simulink model "Shuttle_Orbiter_FDM"  (R2013b)
settings: Solver=ode45  StartTime=0.0  StopTime=1000  RelTol=1e-3
values from neighbouring files (symbols this model uses):
  b = 23.79    [Orbite_InitialParamaters.m]
  c = 12.06    [Orbite_InitialParamaters.m]
  CD_alpha_mach = [0.11425	0.11975	0.13521	0.16 ... (first row only)    [Aerodynamics.m]
  CD_dbf = [0.0135	0.00959	0.0059	0.00242	-0.0005	0.00005	0.0006	0.0006 ... (first row only)    [Aerodynamics.m]
  CD_de = [0.1526	0.113	0.0796	0.0499	0.0176	-0.0262	-0.0837	-0.1391 ... (first row only)    [Aerodynamics.m]
  CDda = 0    [Aerodynamics.m]
  CDdr = 0    [Aerodynamics.m]
  CDdsb = 0.1    [Aerodynamics.m]
  CG = [1080.0 0.0 370.0]    [Orbite_InitialParamaters.m]
  CL0 = -0.05    [Aerodynamics.m]
  CL_alpha_mach = [-0.5028	-0.51097	-0.52957	-0.58454	-0.59773	-0.61005	-0.62831	-0.65514	-0.65616 ... (first row only)    [Aerodynamics.m]
  Cl_beta = [  0	0	0	0	0	0	0	0 ... (first row only)    [Aerodynamics.m]
  CLalpha = 0.05    [Aerodynamics.m]
  CLalphadot = 0    [Aerodynamics.m]
  Clbeta = -0.001    [Aerodynamics.m]
  Clda = 0.0001    [Aerodynamics.m]
  CLde = 0.02    [Aerodynamics.m]
  CLdf = 0.003    [Aerodynamics.m]
  Cldr = 0.00002    (= 2e-05)    [Aerodynamics.m]
  Cldsb = 0.000008    (= 8e-06)    [Aerodynamics.m]
  Clp = -0.003    [Aerodynamics.m]
  CLq = 0    [Aerodynamics.m]
  Clr = 0.006    [Aerodynamics.m]
  Cm0 = 0.036    [Aerodynamics.m]
  Cma = -0.012    [Aerodynamics.m]
  Cmde = -0.087    [Aerodynamics.m]
  Cmdf = -0.0017    [Aerodynamics.m]
  Cmdsb = 0.006    [Aerodynamics.m]
  Cmq = 0.058    [Aerodynamics.m]
  Cnbeta = 0.0016    [Aerodynamics.m]
  Cnda = 0.00005    (= 5e-05)    [Aerodynamics.m]
  Cndr = 0.000006    (= 6e-06)    [Aerodynamics.m]
  Cndsb = 0    [Aerodynamics.m]
  Cnp = -0.0046    [Aerodynamics.m]
  Cnr = -0.005    [Aerodynamics.m]
  CP = [1080.0 0.0 370.0]    [Orbite_InitialParamaters.m]
  CY_da = [0.00106	0.00048 	-0.00002	-0.0005     -0.0008 	-0.00102	-0.00116	-0.0014     -0.00125 ... (first row only)    [Aerodynamics.m]
  CY_de = [  -0.0004	0        0.0004	0.00096	0.0012	0.00111	0.0007	0.00045 ... (first row only)    [Aerodynamics.m]
  CY_dr = [   0.00315	0.0031	0.003	0.0029	0.00275	0.00262	0.0026	0.0026 ... (first row only)    [Aerodynamics.m]
  CY_dsb = [  0.00015 0.00007 0.00015 0.0004 0.0008	0.00133	0.002	0.0026 ... (first row only)    [Aerodynamics.m]
  CYbeta = -0.02    [Aerodynamics.m]
  CYda = 0.003    [Aerodynamics.m]
  CYdr = -0.00002    (= -2e-05)    [Aerodynamics.m]
  CYp = 0    [Aerodynamics.m]
  CYr = 0    [Aerodynamics.m]
  GlideSlopeInitial = -20    [Orbite_InitialParamaters.m]
  h_Initial = 3187+0    (= 3187)    [Orbite_InitialParamaters.m]
  heading0 = 117.5    [Orbite_InitialParamaters.m]
  HglideOrbiter = GligeSlope(:,2)    [Orbite_InitialParamaters.m]
  Iyy = 8729397    [Orbite_InitialParamaters.m]
  LongLat0 = [initial_deg(2); initial_deg(1)]    [Orbite_InitialParamaters.m]
  mass = 83000    [Orbite_InitialParamaters.m]
  runway_alt = 1    [Orbite_InitialParamaters.m]
  runway_deg = dms2degrees(runway_dms_FG)    [Orbite_InitialParamaters.m]
  S = 249.91    [Orbite_InitialParamaters.m]
  Tc = 1/25    (= 0.04)    [Orbite_InitialParamaters.m]
  XglideOrbiter = GligeSlope(:,1)    [Orbite_InitialParamaters.m]
undefined symbols (not defined in the file or in its folder): Earth, Receive, Send, WGS84
libraries: aerolibconvert2 x17, aerolibfltsims x5, simulink x3, aerolibasang x3, aerolibtransform2 x2, aerolibobsolete x1, aerolib6dof2 x1, aerolibatmos2 x1, aerolibgravity2 x1
(part 2 of 2)

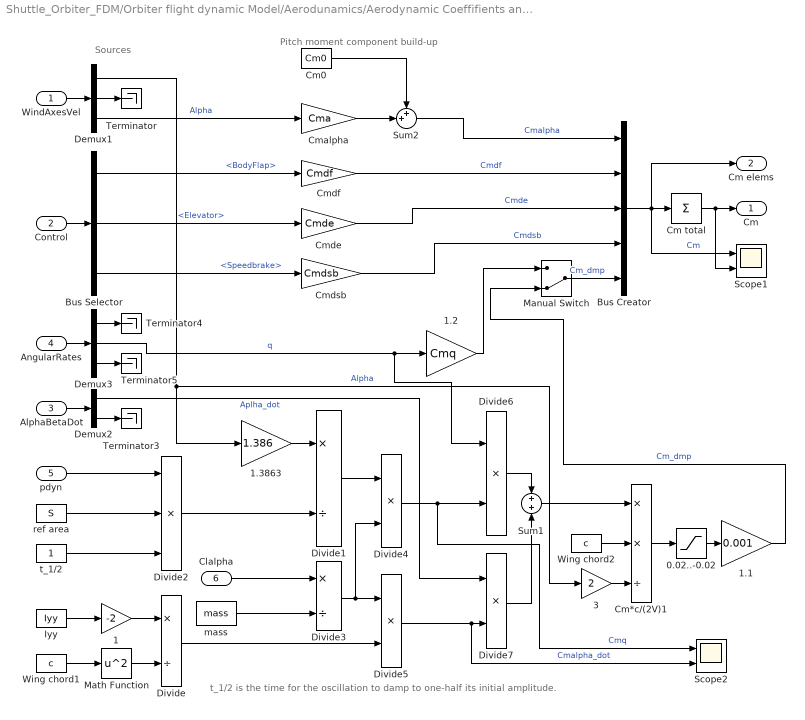
== system Shuttle_Orbiter_FDM/Orbiter flight dynamic Model/Aerodunamics/Aerodynamic Coeffifients and Loads/Pitch Moment Coefficient ==
  note: t_1/2 is the time for the oscillation to damp to one-half its initial amplitude.
  note: Sources
  note: Pitch moment component build-up
  WindAxesVel : Inport
  Control : Inport  Port=2
  AlphaBetaDot : Inport  Port=3
  AngularRates : Inport  Port=4
  pdyn : Inport  Port=5
  Clalpha : Inport  Port=6
  0.02..-0.02 : Saturate  UpperLimit=0.02  LowerLimit=-0.02
  1 : Gain  Gain=-2  SaturateOnIntegerOverflow=on  OutDataTypeStr=Inherit: Same as input  ParamDataTypeStr=Inherit: Same as input
  1.1 : Gain  Gain=0.001  SaturateOnIntegerOverflow=on  OutDataTypeStr=Inherit: Same as input  ParamDataTypeStr=Inherit: Same as input
  1.2 : Gain  Gain=Cmq  SaturateOnIntegerOverflow=on  OutDataTypeStr=Inherit: Same as input  ParamDataTypeStr=Inherit: Same as input
  1.3863 : Gain  Gain=1.386  SaturateOnIntegerOverflow=on  OutDataTypeStr=Inherit: Same as input  ParamDataTypeStr=Inherit: Same as input
  3 : Gain  Gain=2  SaturateOnIntegerOverflow=on  OutDataTypeStr=Inherit: Same as input  ParamDataTypeStr=Inherit: Same as input
  Bus Creator : BusCreator  Inputs=5
  Bus Selector : BusSelector  OutputSignals=BodyFlap,Elevator,Speedbrake
  Cm total : Sum  Inputs=+
  Cm*c/(2V)1 : Product  Inputs=**/  SaturateOnIntegerOverflow=on  InputSameDT=on  OutDataTypeStr=Inherit: Same as first input
  Cm0 : Constant  Value=Cm0  SampleTime=Tc
  Cmalpha : Gain  Gain=Cma  SaturateOnIntegerOverflow=on  OutDataTypeStr=Inherit: Same as input  ParamDataTypeStr=Inherit: Same as input
  Cmde : Gain  Gain=Cmde  SaturateOnIntegerOverflow=on  OutDataTypeStr=Inherit: Same as input  ParamDataTypeStr=Inherit: Same as input
  Cmdf : Gain  Gain=Cmdf  SaturateOnIntegerOverflow=on  OutDataTypeStr=Inherit: Same as input  ParamDataTypeStr=Inherit: Same as input
  Cmdsb : Gain  Gain=Cmdsb  SaturateOnIntegerOverflow=on  OutDataTypeStr=Inherit: Same as input  ParamDataTypeStr=Inherit: Same as input
  Demux1 : Demux  Outputs=3
  Demux2 : Demux  Outputs=2
  Demux3 : Demux  Outputs=3
  Divide : Product  Inputs=*/
  Divide1 : Product  Inputs=*/
  Divide2 : Product  Inputs=3
  Divide3 : Product  Inputs=*/
  Divide{4..7} (4 alike) : Product  Inputs=**
  Iyy : Constant  Value=Iyy  SampleTime=Tc
  Manual Switch : ManualSwitch  CurrentSetting=0
  Math Function : Math  Operator=square  SaturateOnIntegerOverflow=on
  Scope1 : Scope  NumInputPorts=2
      settings: ShowLegends=on  YMin=-0.003~-0.003  YMax=0.003~0.003
  Scope2 : Scope  NumInputPorts=2
      settings: ShowLegends=on  YMin=2.6e-11~-0.0715  YMax=2.925e-11~-0.064  SaveName=ScopeData2
  Sum1 : Sum  SaturateOnIntegerOverflow=on  InputSameDT=on  OutDataTypeStr=Inherit: Same as first input
  Sum2 : Sum  Inputs=++|  SaturateOnIntegerOverflow=on  InputSameDT=on  OutDataTypeStr=Inherit: Same as first input
  Terminator{,3..5} (4 alike) : Terminator
  Wing chord1 : Constant  Value=c  SampleTime=Tc
  Wing chord2 : Constant  Value=c  SampleTime=Tc
  mass : Constant  Value=mass  SampleTime=Tc
  ref area : Constant  Value=S  SampleTime=Tc
  t_1/2 : Constant  SampleTime=Tc
  Cm : Outport
  Cm elems : Outport  Port=2
  wires:
  WindAxesVel/1 -> Demux1/1
  Demux1/1 -> 1.3863/1, 3/1  "Alpha"
  Demux1/2 -> Terminator/1
  Demux1/3 -> Cmalpha/1  "Alpha"
  Control/1 -> Bus Selector/1
  Demux2/1 -> Divide7/1  "Aplha_dot"
  Demux2/2 -> Terminator3/1
  AlphaBetaDot/1 -> Demux2/1
  AngularRates/1 -> Demux3/1
  Demux3/1 -> Terminator4/1
  Demux3/2 -> Divide6/1, 1.2/1  "q"
  Demux3/3 -> Terminator5/1
  Cm0/1 -> Sum2/1
  Cmalpha/1 -> Sum2/2
  Cmdf/1 -> Bus Creator/2  "Cmdf"
  Cmde/1 -> Bus Creator/3  "Cmde"
  Bus Selector/1 -> Cmdf/1  "<BodyFlap>"
  Bus Selector/2 -> Cmde/1  "<Elevator>"
  Bus Selector/3 -> Cmdsb/1  "<Speedbrake>"
  Cmdsb/1 -> Bus Creator/4  "Cmdsb"
  Bus Creator/1 -> Scope1/1, Cm total/1, Cm elems/1  "Cm"
  Iyy/1 -> 1/1
  Wing chord1/1 -> Math Function/1
  1/1 -> Divide/1
  Math Function/1 -> Divide/2
  1.3863/1 -> Divide1/1
  pdyn/1 -> Divide2/1
  ref area/1 -> Divide2/2
  t_1/2/1 -> Divide2/3
  Divide2/1 -> Divide1/2
  mass/1 -> Divide3/2
  Divide/1 -> Divide5/2
  Divide1/1 -> Divide4/1
  0.02..-0.02/1 -> 1.1/1
  Cm total/1 -> Scope1/2, Cm/1
  Divide3/1 -> Divide4/2, Divide5/1
  Divide4/1 -> Scope2/1, Divide6/2  "Cmq"
  Divide5/1 -> Scope2/2, Divide7/2  "Cmalpha_dot"
  Divide7/1 -> Sum1/2
  Divide6/1 -> Sum1/1
  3/1 -> Cm*c/(2V)1/3
  Wing chord2/1 -> Cm*c/(2V)1/2
  Sum1/1 -> Cm*c/(2V)1/1
  Cm*c/(2V)1/1 -> 0.02..-0.02/1
  Sum2/1 -> Bus Creator/1  "Cmalpha"
  1.1/1 -> Manual Switch/2  "Cm_dmp"
  Clalpha/1 -> Divide3/1
  Manual Switch/1 -> Bus Creator/5  "Cm_dmp"
  1.2/1 -> Manual Switch/1

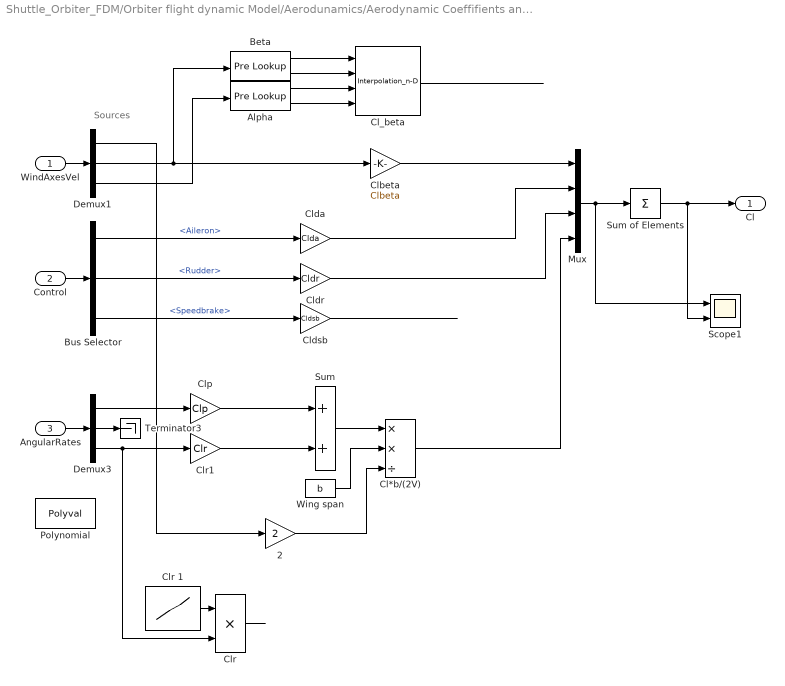
== system Shuttle_Orbiter_FDM/Orbiter flight dynamic Model/Aerodunamics/Aerodynamic Coeffifients and Loads/Roll Moment Coefficient ==
  note: Sources
  WindAxesVel : Inport
  Control : Inport  Port=2
  AngularRates : Inport  Port=3
  2 : Gain  Gain=2  SaturateOnIntegerOverflow=on  OutDataTypeStr=Inherit: Same as input  ParamDataTypeStr=Inherit: Same as input
  Alpha : PreLookup  BreakpointsData=|  ExtrapMethod=Linear
      | [-10 -5  0	5 10  15 20 25
      | ]
  Beta : PreLookup  BreakpointsData=|  ExtrapMethod=Linear
      | [0
      | 1
      | 2
      | 4
      | 6
      | 8
      | 10
      | ]
  Bus Selector : BusSelector  OutputSignals=Aileron,Rudder,Speedbrake
  Cl*b/(2V) : Product  Inputs=**/  SaturateOnIntegerOverflow=on  InputSameDT=on  OutDataTypeStr=Inherit: Same as first input
  "Cl_beta " : Interpolation_n-D  Table=Cl_beta  InternalRulePriority=Speed
  Clbeta : Gain  Gain=Clbeta  SaturateOnIntegerOverflow=on  OutDataTypeStr=Inherit: Same as input  ParamDataTypeStr=Inherit: Same as input
  Clda : Gain  Gain=Clda  SaturateOnIntegerOverflow=on  OutDataTypeStr=Inherit: Same as input  ParamDataTypeStr=Inherit: Same as input
  Cldr : Gain  Gain=Cldr  SaturateOnIntegerOverflow=on  OutDataTypeStr=Inherit: Same as input  ParamDataTypeStr=Inherit: Same as input
  Cldsb : Gain  Gain=Cldsb  SaturateOnIntegerOverflow=on  OutDataTypeStr=Inherit: Same as input  ParamDataTypeStr=Inherit: Same as input
  Clp : Gain  Gain=Clp  SaturateOnIntegerOverflow=on  OutDataTypeStr=Inherit: Same as input  ParamDataTypeStr=Inherit: Same as input
  Clr : Product  SaturateOnIntegerOverflow=on  InputSameDT=on  OutDataTypeStr=Inherit: Same as first input
  Clr 1 : Lookup_n-D  NumberOfTableDimensions=1  BreakpointsForDimension1=|  Table=|  InternalRulePriority=Speed  RndMeth=Simplest  InputSameDT=on
      BreakpointsForDimension1=|
      | [0
      | 10
      | 20
      | 30
      | 40
      | 50
      | ]
      Table=|
      | [0.125
      | 0.188
      | 0.225
      | 0.1
      | 0.075
      | 0.007
      | ]
  Clr1 : Gain  Gain=Clr  SaturateOnIntegerOverflow=on  OutDataTypeStr=Inherit: Same as input  ParamDataTypeStr=Inherit: Same as input
  Demux1 : Demux  Outputs=3
  Demux3 : Demux  Outputs=3
  Mux : Mux
  Polynomial : Polyval  Coefs=[ +2.081618890e-019, -1.441693666e-014, +4.719686976e-010, -8.536869453e-006, +1.621573104e-001, -8.087801117e+001 ]
  Scope1 : Scope  NumInputPorts=2
      settings: ShowLegends=on  YMin=-0.005~-0.005  YMax=0.008~0.008  SaveName=ScopeData3
  Sum : Sum  SaturateOnIntegerOverflow=on  InputSameDT=on  OutDataTypeStr=Inherit: Same as first input
  Sum of Elements : Sum  Inputs=+
  Terminator3 : Terminator
  Wing span : Constant  Value=b  SampleTime=Tc
  Cl : Outport
  wires:
  Clp/1 -> Sum/1
  Clr/1 -> ?
  Sum/1 -> Cl*b/(2V)/1
  Wing span/1 -> Cl*b/(2V)/2
  WindAxesVel/1 -> Demux1/1
  Demux1/1 -> 2/1
  Demux1/2 -> Beta/1, Clbeta/1
  Demux1/3 -> Alpha/1
  AngularRates/1 -> Demux3/1
  Demux3/1 -> Clp/1
  Demux3/2 -> Terminator3/1
  Demux3/3 -> Clr1/1, Clr/2
  Clbeta/1 -> Mux/1
  Clda/1 -> Mux/2
  Cldr/1 -> Mux/3
  Cl*b/(2V)/1 -> Mux/4
  2/1 -> Cl*b/(2V)/3
  Control/1 -> Bus Selector/1
  Bus Selector/1 -> Clda/1  "<Aileron>"
  Bus Selector/2 -> Cldr/1  "<Rudder>"
  Alpha/1 -> "Cl_beta "/3
  Alpha/2 -> "Cl_beta "/4
  Beta/1 -> "Cl_beta "/1
  Beta/2 -> "Cl_beta "/2
  "Cl_beta "/1 -> ?
  Bus Selector/3 -> Cldsb/1  "<Speedbrake>"
  Cldsb/1 -> ?
  Clr1/1 -> Sum/2
  Clr 1/1 -> Clr/1
  Mux/1 -> Sum of Elements/1, Scope1/1
  Sum of Elements/1 -> Cl/1, Scope1/2

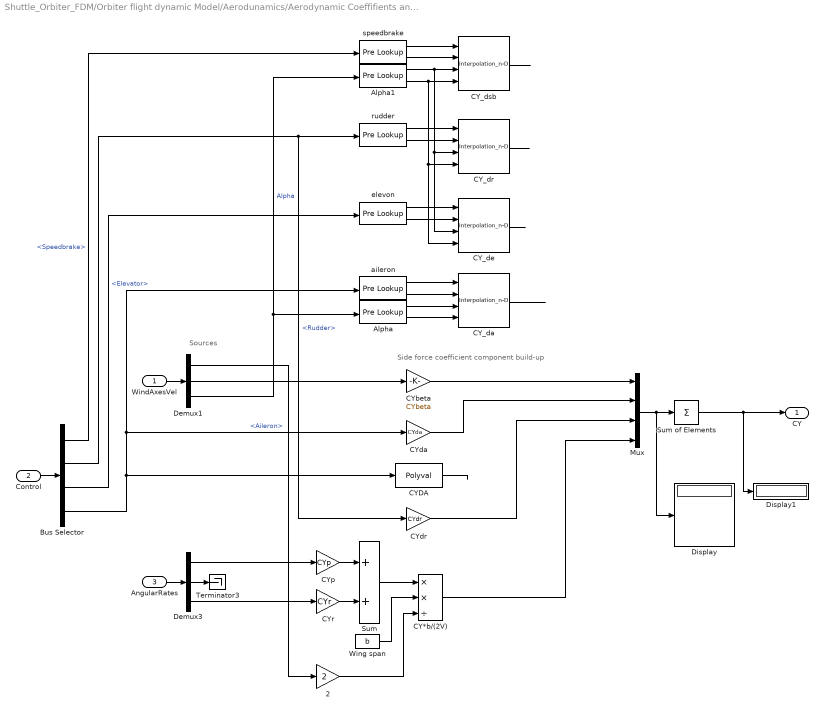
== system Shuttle_Orbiter_FDM/Orbiter flight dynamic Model/Aerodunamics/Aerodynamic Coeffifients and Loads/Side Force Coefficient ==
  note: Sources
  note: Side force coefficient component build-up
  WindAxesVel : Inport
  Control : Inport  Port=2
  AngularRates : Inport  Port=3
  2 : Gain  Gain=2  SaturateOnIntegerOverflow=on  OutDataTypeStr=Inherit: Same as input  ParamDataTypeStr=Inherit: Same as input
  Alpha : PreLookup  BreakpointsData=|  ExtrapMethod=Linear
      | [-10 -5  0	5 10 13 15 20 25
      | ]
  Alpha1 : PreLookup  BreakpointsData=|  ExtrapMethod=Linear
      | [-10 -5  0	5 10  15 20 25
      | ]
  Bus Selector : BusSelector  OutputSignals=Speedbrake,Rudder,Elevator,Aileron
  CY*b/(2V) : Product  Inputs=**/  SaturateOnIntegerOverflow=on  InputSameDT=on  OutDataTypeStr=Inherit: Same as first input
  "CYDA " : Polyval  Coefs=[0.000004 000001 -0.004]
  CY_da : Interpolation_n-D  Table=CY_da  InternalRulePriority=Speed
  CY_de : Interpolation_n-D  Table=CY_de  InternalRulePriority=Speed
  CY_dr : Interpolation_n-D  Table=CY_dr  InternalRulePriority=Speed
  CY_dsb : Interpolation_n-D  Table=CY_dsb  InternalRulePriority=Speed
  CYbeta : Gain  Gain=CYbeta  SaturateOnIntegerOverflow=on  OutDataTypeStr=Inherit: Same as input  ParamDataTypeStr=Inherit: Same as input
  "CYda " : Gain  Gain=CYda  SaturateOnIntegerOverflow=on  OutDataTypeStr=Inherit: Same as input  ParamDataTypeStr=Inherit: Same as input
  CYdr : Gain  Gain=CYdr  SaturateOnIntegerOverflow=on  OutDataTypeStr=Inherit: Same as input  ParamDataTypeStr=Inherit: Same as input
  CYp : Gain  Gain=CYp  SaturateOnIntegerOverflow=on  OutDataTypeStr=Inherit: Same as input  ParamDataTypeStr=Inherit: Same as input
  CYr : Gain  Gain=CYr  SaturateOnIntegerOverflow=on  OutDataTypeStr=Inherit: Same as input  ParamDataTypeStr=Inherit: Same as input
  Demux1 : Demux  Outputs=3
  Demux3 : Demux  Outputs=3
  Display : Display
  Display1 : Display
  Mux : Mux
  Sum : Sum  SaturateOnIntegerOverflow=on  InputSameDT=on  OutDataTypeStr=Inherit: Same as first input
  Sum of Elements : Sum  Inputs=+
  Terminator3 : Terminator
  Wing span : Constant  Value=b  SampleTime=Tc
  aileron : PreLookup  BreakpointsData=|  ExtrapMethod=Linear
      | [-30
      | -25
      | -20
      | -15
      | -10
      | -5
      | 0
      | 5
      | 10
      | 15]
  elevon : PreLookup  BreakpointsData=|  ExtrapMethod=Linear
      | [-30
      | -25
      | -20
      | -15
      | -10
      | -5
      | 0
      | 5
      | 10
      | 15
      | ]
  rudder : PreLookup  BreakpointsData=|  ExtrapMethod=Linear
      | [0
      | 7.5
      | 15
      | 25
      | 35
      | 45
      | 55
      | 70
      | 87.2
      | ]
  speedbrake : PreLookup  BreakpointsData=|  ExtrapMethod=Linear
      | [0
      | 15
      | 25
      | 35
      | 45
      | 55
      | 70
      | 87.2
      | ]
  CY : Outport
  wires:
  CYp/1 -> Sum/1
  CYr/1 -> Sum/2
  Sum/1 -> CY*b/(2V)/1
  Wing span/1 -> CY*b/(2V)/2
  WindAxesVel/1 -> Demux1/1
  Demux1/1 -> 2/1
  Demux1/2 -> CYbeta/1
  Control/1 -> Bus Selector/1
  AngularRates/1 -> Demux3/1
  Demux3/1 -> CYp/1
  Demux3/2 -> Terminator3/1
  Demux3/3 -> CYr/1
  CYbeta/1 -> Mux/1
  "CYda "/1 -> Mux/2
  CYdr/1 -> Mux/3
  CY*b/(2V)/1 -> Mux/4
  Sum of Elements/1 -> Display1/1, CY/1
  2/1 -> CY*b/(2V)/3
  Alpha/1 -> CY_da/3
  aileron/1 -> CY_da/1
  aileron/2 -> CY_da/2
  Alpha/2 -> CY_da/4
  CY_da/1 -> ?
  Bus Selector/4 -> "CYDA "/1, aileron/1, "CYda "/1  "<Aileron>"
  Alpha1/1 -> CY_de/3, CY_dr/3, CY_dsb/3
  elevon/1 -> CY_de/1
  elevon/2 -> CY_de/2
  Alpha1/2 -> CY_dsb/4, CY_de/4, CY_dr/4
  Bus Selector/3 -> elevon/1  "<Elevator>"
  CY_de/1 -> ?
  Demux1/3 -> Alpha/1, Alpha1/1  "Alpha"
  rudder/1 -> CY_dr/1
  rudder/2 -> CY_dr/2
  Bus Selector/2 -> CYdr/1, rudder/1  "<Rudder>"
  CY_dr/1 -> ?
  speedbrake/1 -> CY_dsb/1
  speedbrake/2 -> CY_dsb/2
  Bus Selector/1 -> speedbrake/1  "<Speedbrake>"
  CY_dsb/1 -> ?
  "CYDA "/1 -> ?
  Mux/1 -> Display/1, Sum of Elements/1

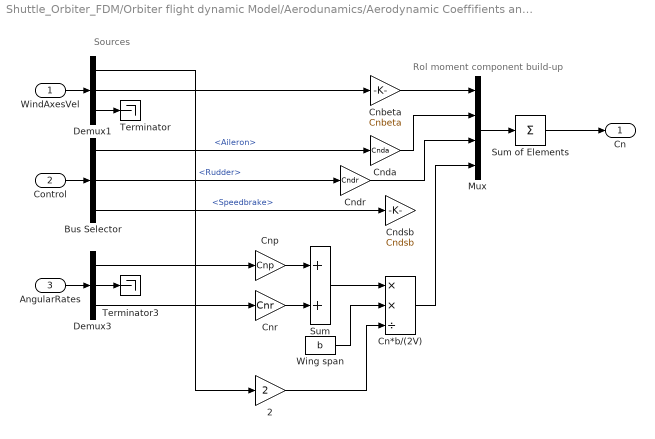
== system Shuttle_Orbiter_FDM/Orbiter flight dynamic Model/Aerodunamics/Aerodynamic Coeffifients and Loads/Yaw Moment Coefficient  ==
  note: Rol moment component build-up
  note: Sources
  WindAxesVel : Inport
  Control : Inport  Port=2
  AngularRates : Inport  Port=3
  2 : Gain  Gain=2  SaturateOnIntegerOverflow=on  OutDataTypeStr=Inherit: Same as input  ParamDataTypeStr=Inherit: Same as input
  Bus Selector : BusSelector  OutputSignals=Aileron,Rudder,Speedbrake
  Cn*b/(2V) : Product  Inputs=**/  SaturateOnIntegerOverflow=on  InputSameDT=on  OutDataTypeStr=Inherit: Same as first input
  Cnbeta : Gain  Gain=Cnbeta  SaturateOnIntegerOverflow=on  OutDataTypeStr=Inherit: Same as input  ParamDataTypeStr=Inherit: Same as input
  Cnda : Gain  Gain=Cnda  SaturateOnIntegerOverflow=on  OutDataTypeStr=Inherit: Same as input  ParamDataTypeStr=Inherit: Same as input
  Cndr : Gain  Gain=Cndr  SaturateOnIntegerOverflow=on  OutDataTypeStr=Inherit: Same as input  ParamDataTypeStr=Inherit: Same as input
  Cndsb : Gain  Gain=Cndsb  SaturateOnIntegerOverflow=on  OutDataTypeStr=Inherit: Same as input  ParamDataTypeStr=Inherit: Same as input
  Cnp : Gain  Gain=Cnp  SaturateOnIntegerOverflow=on  OutDataTypeStr=Inherit: Same as input  ParamDataTypeStr=Inherit: Same as input
  Cnr : Gain  Gain=Cnr  SaturateOnIntegerOverflow=on  OutDataTypeStr=Inherit: Same as input  ParamDataTypeStr=Inherit: Same as input
  Demux1 : Demux  Outputs=3
  Demux3 : Demux  Outputs=3
  Mux : Mux
  Sum : Sum  SaturateOnIntegerOverflow=on  InputSameDT=on  OutDataTypeStr=Inherit: Same as first input
  Sum of Elements : Sum  Inputs=+
  Terminator : Terminator
  Terminator3 : Terminator
  Wing span : Constant  Value=b  SampleTime=Tc
  Cn : Outport
  wires:
  Sum of Elements/1 -> Cn/1
  Cndr/1 -> Mux/3
  Cnda/1 -> Mux/2
  Cnbeta/1 -> Mux/1
  Demux3/3 -> Cnr/1
  Demux3/2 -> Terminator3/1
  Demux3/1 -> Cnp/1
  AngularRates/1 -> Demux3/1
  Control/1 -> Bus Selector/1
  Demux1/3 -> Terminator/1
  Demux1/2 -> Cnbeta/1
  Demux1/1 -> 2/1
  WindAxesVel/1 -> Demux1/1
  Wing span/1 -> Cn*b/(2V)/2
  Sum/1 -> Cn*b/(2V)/1
  Cnr/1 -> Sum/2
  Cnp/1 -> Sum/1
  2/1 -> Cn*b/(2V)/3
  Cn*b/(2V)/1 -> Mux/4
  Bus Selector/1 -> Cnda/1  "<Aileron>"
  Bus Selector/2 -> Cndr/1  "<Rudder>"
  Bus Selector/3 -> Cndsb/1  "<Speedbrake>"
  Mux/1 -> Sum of Elements/1
